simulink model "ex2"  (R2016a)
settings: Solver=VariableStepAuto  StartTime=0.0  StopTime=10.0  RelTol=1e-3

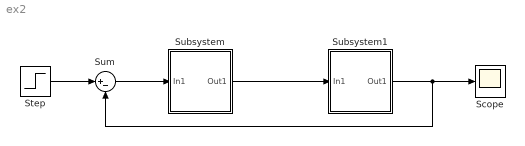
== system ex2 ==
  Scope : Scope
  Step : Step  SampleTime=0
  Subsystem : Subsystem  mask{b=3}
      mask Callback b:
      | if str2num(get_param(gcb,'b'))<0
      |     error('nr este negativ')
      | end
  Subsystem1 : Subsystem  mask{kp=3, ki=7}
      mask prompts: kp "param1"; ki "param2"
      mask Callback kp:
      | if str2num(get_param(gcb,'kp'))<0
      |     error('nr negativ')
      | end
      mask Callback ki:
      | if str2num(get_param(gcb,'ki'))<0
      |     error('nr negativ')
      | end
  Sum : Sum  Inputs=|+-
  wires:
  Step/1 -> Sum/1
  Sum/1 -> Subsystem/1(In1)
  Subsystem1/1(Out1) -> Sum/2, Scope/1
  Subsystem/1(Out1) -> Subsystem1/1(In1)

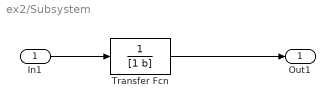
== system ex2/Subsystem ==
  In1 : Inport
  Transfer Fcn : TransferFcn  Denominator=[1 b]
  Out1 : Outport
  wires:
  Transfer Fcn/1 -> Out1/1
  In1/1 -> Transfer Fcn/1

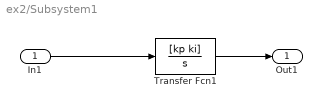
== system ex2/Subsystem1 ==
  In1 : Inport
  Transfer Fcn1 : TransferFcn  Numerator=[kp ki]  Denominator=[1 0]
  Out1 : Outport
  wires:
  In1/1 -> Transfer Fcn1/1
  Transfer Fcn1/1 -> Out1/1
